simulink model "mcb_pmsm_foc_hall_f28379d_state_indicator"  (R2023b)
settings: Solver=FixedStepDiscrete  StartTime=0.0  StopTime=8  RelTol=1e-3  EnableMultiTasking=on
InitFcn:
  | mcb_pmsm_foc_hall_f28379d_data;
model workspace (MAT data in the model file):
  encoderResolution = 2000
  hallOffset = '0.5'
  indexOffset = 850
  polePairs = '4'
values from neighbouring files (symbols this model uses):
  dataType = 'single'    [mcb_pmsm_foc_hall_f28069m_data.m]    (also in mcb_pmsm_foc_hall_f28379d_data.m)
  inverter = mcb_SetInverterParameters('DRV8312-C2-KIT')    [mcb_pmsm_foc_hall_f28069m_data.m]    (also in mcb_pmsm_foc_hall_f28379d_data.m = mcb_updateInverterParameters(pmsm,inverter,target))
  PI_params = mcb_SetControllerParameters(pmsm,inverter,PU_System,T_pwm,Ts,Ts_speed)    [mcb_pmsm_foc_hall_f28069m_data.m]    (also in mcb_pmsm_foc_hall_f28379d_data.m)
  pmsm = mcb_SetPMSMMotorParameters('BLY171D')    [mcb_pmsm_foc_hall_f28069m_data.m]    (also in mcb_pmsm_foc_hall_f28379d_data.m = mcb_SetPMSMMotorParameters('custom'))
  PU_System = mcb_SetPUSystem(pmsm,inverter)    [mcb_pmsm_foc_hall_f28069m_data.m]    (also in mcb_pmsm_foc_hall_f28379d_data.m)
  target = mcb_SetProcessorDetails('F28069M',PWM_frequency)    [mcb_pmsm_foc_hall_f28069m_data.m]    (also in mcb_pmsm_foc_hall_f28379d_data.m = mcb_SetProcessorDetails('F28379D',PWM_frequency))
  Ts = T_pwm    (= 5e-05)    [mcb_pmsm_foc_hall_f28069m_data.m]    (also in mcb_pmsm_foc_hall_f28379d_data.m)
  Ts_motor = T_pwm/2    (= 2.5e-05)    [mcb_pmsm_foc_hall_f28069m_data.m]    (also in mcb_pmsm_foc_hall_f28379d_data.m)
  Ts_simulink = T_pwm/2    (= 2.5e-05)    [mcb_pmsm_foc_hall_f28069m_data.m]    (also in mcb_pmsm_foc_hall_f28379d_data.m)
  Ts_speed = 10*Ts    (= 0.0005)    [mcb_pmsm_foc_hall_f28069m_data.m]    (also in mcb_pmsm_foc_hall_f28379d_data.m)
undefined symbols (not defined in the file or in its folder): DiscIntNeverNeededParam, Down, GPTRIP1SEL, GPTRIP2SEL, Ts_sensor, TZ1, TZ2, Up
libraries: simulink x37, mcbpositiondecoderlib x12, mcbcontrolslib x11, idelinklib_common x8, c280xlib x8, c2802xlib x7, svdschedulerlib x5, slpidlib x4, c2837xDlib x3, dspfdesign x2, cstblocks x2, svdutilitieslib x1
(part 1 of 4)
settings Model: ExtModeTrigDuration=8  Creator=The MathWorks, Inc.  LastModifiedBy=13571
settings SolverCC: AlgebraicLoopSolver=TrustRegion  AutoInsertRateTranBlk=on
settings DataIOCC: LimitDataPoints=on  SaveFormat=Array  SaveOutput=off  SaveTime=off  ReturnWorkspaceOutputs=off
settings OptimizationCC: DefaultParameterBehavior=Inlined  DefaultUnderspecifiedDataType=single  OptimizeBlockIOStorage=off  BufferReuse=off  ReuseModelBlockBuffer=off  GlobalBufferReuse=off  ExpressionFolding=off  ExpressionDepthLimit=2147483647  LocalBlockOutputs=off  InitFltsAndDblsToZero=on  NoFixptDivByZeroProtection=on  EfficientFloat2IntCast=on  EfficientMapNaN2IntZero=off  LifeSpan=Inf  MaxStackSize=512  OptimizeDataStoreBuffers=off  BusAssignmentInplaceUpdate=off  EfficientTunableParamExpr=on
settings DebuggingCC: ReadBeforeWriteMsg=DisableAll  WriteAfterWriteMsg=DisableAll  WriteAfterReadMsg=DisableAll  CheckSSInitialOutputMsg=off  SignalResolutionControl=TryResolveAllWithWarning  SolverPrmCheckMsg=warning  InheritedTsInSrcMsg=none  MultiTaskDSMMsg=none  MultiTaskCondExecSysMsg=none  TasksWithSamePriorityMsg=none  SigSpecEnsureSampleTimeMsg=none  IntegerOverflowMsg=none  ParameterPrecisionLossMsg=none  FcnCallInpInsideContextMsg=warning  UnconnectedInputMsg=warning  UnconnectedOutputMsg=warning  UnconnectedLineMsg=warning  AllowSymbolicDim=off  StateNameClashWarn=warning  PregeneratedLibrarySubsystemCodeDiagnostic=none  SFUnexpectedBacktrackingDiag=warning  SFNoUnconditionalDefaultTransitionDiag=warning  SFExecutionAtInitializationDiag=none  IntegerSaturationMsg=none  ArithmeticOperatorsInVariantConditions=warning
settings HardwareCC: ProdBitPerChar=16  ProdBitPerInt=16  ProdBitPerPointer=32  ProdBitPerSizeT=32  ProdBitPerPtrDiffT=32  ProdLargestAtomicInteger=Integer  ProdLargestAtomicFloat=None  ProdWordSize=16  ProdLongLongMode=on  ProdHWDeviceType=Texas Instruments->C2000  TargetBitPerChar=16  TargetBitPerInt=16  TargetBitPerPointer=16  TargetLargestAtomicInteger=Integer  TargetIntDivRoundTo=Zero  TargetEndianess=LittleEndian  TargetWordSize=16  TargetHWDeviceType=TI C2000
settings ModelReferenceCC: EnableRefExpFcnMdlSchedulingChecks=on  PropagateSignalLabelsOutOfModel=off
settings SFSimCC: SimUseLocalCustomCode=off  MATLABDynamicMemAlloc=off
settings RTWCC: Description=Embedded Coder  SystemTargetFile=ert.tlc  HardwareBoard=TI Delfino F28379D LaunchPad  TemplateMakefile=ert_default_tmf  GenerateReport=on  RTWUseLocalCustomCode=off  Toolchain=Texas Instruments Code Composer Studio (C2000)  IncludeHyperlinkInReport=on  GenerateTraceInfo=on  GenerateTraceReport=on  GenerateTraceReportSl=on  GenerateTraceReportSf=on  GenerateTraceReportEml=on  DLArmComputeVersion=19.05
settings CodeAppCC: IgnoreCustomStorageClasses=off  CustomSymbolStrType=$N$R$M  StateflowObjectComments=on  InternalIdentifier=Classic
settings ERTTargetCC: CodeReplacementLibrary=TI C28x  MultiwordLength=2048  ConvertIfToSwitch=off  SuppressUnreachableDefaultCases=off  MemSecPackage=tic2000demospkg
settings ConfigComp: CovMetricSettings=dw  CovSaveCumulativeToWorkspaceVar=on  CovSaveSingleToWorkspaceVar=on  CovExternalEMLEnable=off  CovSFcnEnable=off

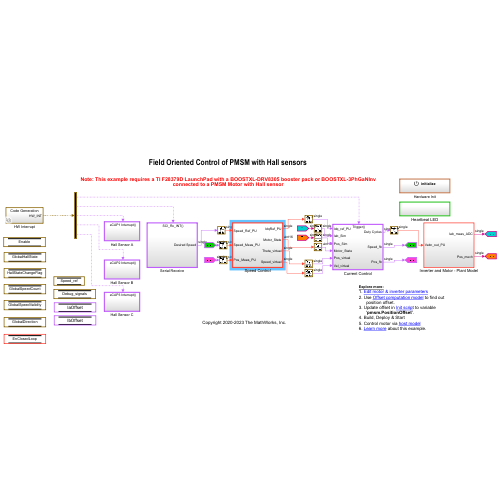
[thumbnail: Simulink's stored preview of the top-level diagram]
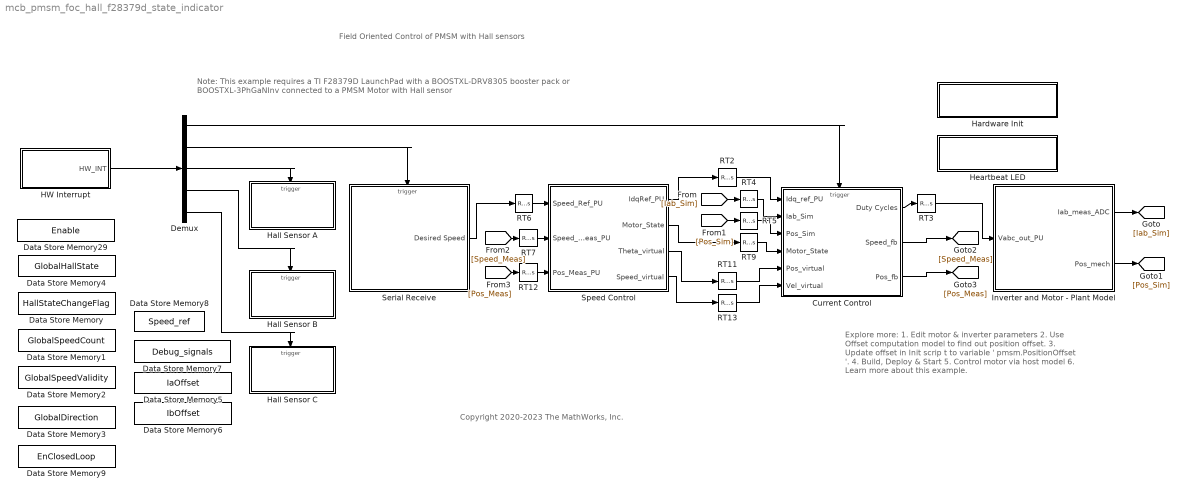
== system mcb_pmsm_foc_hall_f28379d_state_indicator ==
  note: Copyright 2020-2023 The MathWorks, Inc.
  note: Field Oriented Control of PMSM with Hall sensors
  note: Note: This example requires a TI F28379D LaunchPad with a BOOSTXL-DRV8305 booster pack or BOOSTXL-3PhGaNInv
      | connected to a PMSM Motor with Hall sensor
  note: Explore more:
      | 1. Edit motor & inverter parameters
      | 2. Use Offset computation model to find out position offset.
      | 3. Update offset in Init scrip t to variable ' pmsm.PositionOffset '.
      | 4. Build, Deploy & Start
      | 5. Control motor via host model
      | 6. Learn more about this example.
  Current Control : Subsystem
      settings: RTWSystemCode=Nonreusable function
  Data Store Memory : DataStoreMemory  DataStoreName=HallStateChangeFlag  ShowAdditionalParam=off
  Data Store Memory1 : DataStoreMemory  DataStoreName=GlobalSpeedCount  ShowAdditionalParam=off
  Data Store Memory2 : DataStoreMemory  DataStoreName=GlobalSpeedValidity  ShowAdditionalParam=off
  Data Store Memory29 : DataStoreMemory  DataStoreName=Enable  ShowAdditionalParam=off  OutDataTypeStr=boolean
  Data Store Memory3 : DataStoreMemory  DataStoreName=GlobalDirection  ShowAdditionalParam=off
  Data Store Memory4 : DataStoreMemory  DataStoreName=GlobalHallState  ShowAdditionalParam=off  OutDataTypeStr=uint32
  Data Store Memory5 : DataStoreMemory  DataStoreName=IaOffset  InitialValue=inverter.CtSensAOffset  ShowAdditionalParam=off
  Data Store Memory6 : DataStoreMemory  DataStoreName=IbOffset  InitialValue=inverter.CtSensBOffset  ShowAdditionalParam=off
  Data Store Memory7 : DataStoreMemory  DataStoreName=Debug_signals  ReadBeforeWriteMsg=warning  WriteAfterWriteMsg=warning  WriteAfterReadMsg=warning  InitialValue=5  ShowAdditionalParam=off  OutDataTypeStr=uint16
  Data Store Memory8 : DataStoreMemory  DataStoreName=Speed_ref  ReadBeforeWriteMsg=warning  WriteAfterWriteMsg=warning  WriteAfterReadMsg=warning  ShowAdditionalParam=off  OutDataTypeStr=dataType
  Data Store Memory9 : DataStoreMemory  DataStoreName=EnClosedLoop  WriteAfterWriteMsg=warning  ShowAdditionalParam=off
  Demux : Demux  Outputs=5
  HW Interrupt : Subsystem  Variant=on  VariantControlMode=sim codegen switching
  Hall Sensor A : Subsystem
  Hall Sensor B : Subsystem
  Hall Sensor C : Subsystem
  Hardware Init : Subsystem  TreatAsAtomicUnit=on
  Heartbeat LED : Subsystem  TreatAsAtomicUnit=on
  Inverter and Motor - Plant Model : Subsystem
  RT{2..5,9,11,13} (7 alike) : RateTransition  Deterministic=off
  RT12 : RateTransition  Deterministic=off  OutPortSampleTime=Ts_speed
  RT6 : RateTransition  Deterministic=off  OutPortSampleTime=Ts_speed
  RT7 : RateTransition  Deterministic=off  OutPortSampleTime=Ts_speed
  Serial Receive : Subsystem  SystemSampleTime=1e-3
  Speed Control : Subsystem  TreatAsAtomicUnit=on  SystemSampleTime=Ts_speed
  wires:
  [Iab_Sim] -> RT4/1
  Speed Control/1(IdqRef_PU) -> RT2/1
  [Pos_Sim] -> RT5/1
  RT2/1 -> Current Control/1(Idq_ref_PU)
  RT4/1 -> Current Control/2(Iab_Sim)
  RT5/1 -> Current Control/3(Pos_Sim)
  Current Control/1(Duty Cycles) -> RT3/1
  RT3/1 -> Inverter and Motor - Plant Model/1(Vabc_out_PU)
  Inverter and Motor - Plant Model/1(Iab_meas_ADC) -> [Iab_Sim]
  Inverter and Motor - Plant Model/2(Pos_mech) -> [Pos_Sim]
  Demux/2 -> Serial Receive/Trigger
  Demux/1 -> Current Control/Trigger
  HW Interrupt/1(HW_INT) -> Demux/1
  Demux/3 -> Hall Sensor A/Trigger
  Demux/4 -> Hall Sensor B/Trigger
  Demux/5 -> Hall Sensor C/Trigger
  Serial Receive/1(Desired Speed) -> RT6/1
  RT6/1 -> Speed Control/1(Speed_Ref_PU)
  RT7/1 -> Speed Control/2(Speed_Meas_PU)
  Speed Control/2(Motor_State) -> RT9/1
  RT9/1 -> Current Control/4(Motor_State)
  Speed Control/3(Theta_virtual) -> RT11/1
  RT11/1 -> Current Control/5(Pos_virtual)
  Current Control/2(Speed_fb) -> [Speed_Meas]
  [Speed_Meas] -> RT7/1
  Current Control/3(Pos_fb) -> [Pos_Meas]
  RT12/1 -> Speed Control/3(Pos_Meas_PU)
  [Pos_Meas] -> RT12/1
  Speed Control/4(Speed_virtual) -> RT13/1
  RT13/1 -> Current Control/6(Vel_virtual)

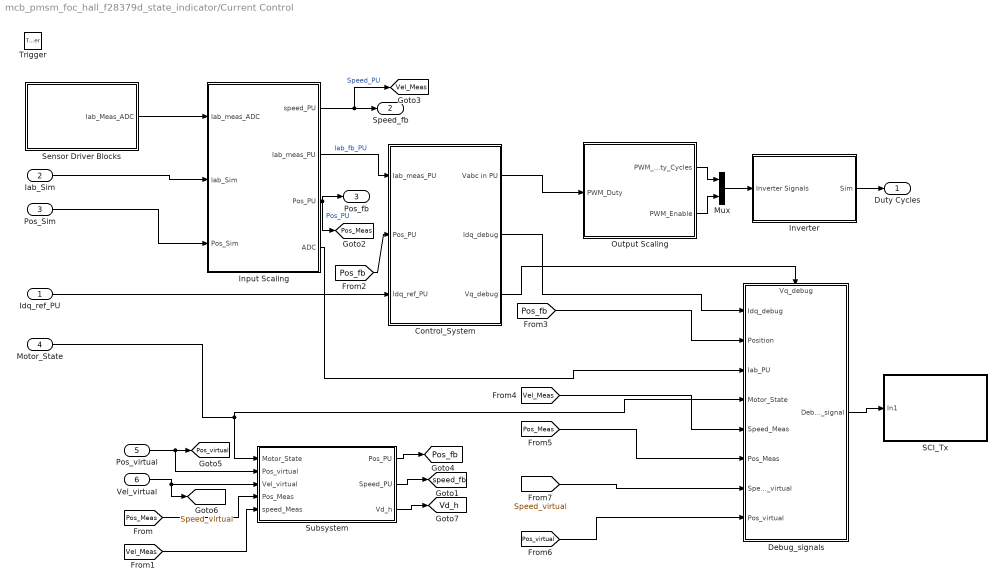
== system mcb_pmsm_foc_hall_f28379d_state_indicator/Current Control ==
  Idq_ref_PU : Inport
  Iab_Sim : Inport  Port=2
  Pos_Sim : Inport  Port=3
  Motor_State : Inport  Port=4
  Pos_virtual : Inport  Port=5
  Vel_virtual : Inport  Port=6
  Trigger : TriggerPort  TriggerType=function-call  VariantControl=Variant  PortDimensions=1
  Control_System : Subsystem
  Debug_signals : Subsystem
      settings: PortSchema="{\"entries\":[{\"content\":{\"sides\":[{\"content\":{\"connectorIds\":[\"In1\",\"In2\",\"In3\",\"In4\",\"In5\",\"In6\",\"In7\",\"In8\"]},\"type\":\"ConnectorPlacement.EquallySpacedRectSide\",\"uuid\":\"67483f5e-56e2-47cf-8de8-9bd8ec9baffc\"},{\"content\":{\"connectorIds\":[\"Out1\"],\"side\":\"RIGHT\"},\"type\":\"ConnectorPlacement.EquallySpacedRectSide\",\"uuid\":\"d939e1f4-c08d-487b-bf48-149d22cc5739\"},{\"content\":{\"connectorIds\":[\"In9\"],\"side\":\"TOP\"},\"type\":\"ConnectorPlacement.EquallySpacedRectSide\",\"uuid\":\"48db4f3d-d2f9-4eaf-b7c1-a7fd508ed9fd\"}]},\"type\":\"ConnectorPlacement.EquallySpacedConnector\",\"uuid\":\"f00bd8a8-e348-4ac0-9697-8b50afb0be3d\"}],\"packageUris\":[\"http://schema.mathworks.com/mf0/Connector/R2020b\"],\"version\":\"1.0\"}"
  Input Scaling : Subsystem  Variant=on  VariantControlMode=sim codegen switching  VariantControl=Variant1  PropagateVariantConditions=on
  Inverter : Subsystem  Variant=on  VariantControlMode=sim codegen switching
  Mux : Mux  Inputs=2
  Output Scaling : Subsystem
  SCI_Tx : Subsystem  Variant=on  VariantControlMode=sim codegen switching
  Sensor Driver Blocks : Subsystem  Variant=on  VariantControlMode=sim codegen switching
  Subsystem : Subsystem
  Duty Cycles : Outport  InitialOutput=0  VectorParamsAs1DForOutWhenUnconnected=off
  Speed_fb : Outport  Port=2  InitialOutput=0  VectorParamsAs1DForOutWhenUnconnected=off
  Pos_fb : Outport  Port=3  InitialOutput=0  VectorParamsAs1DForOutWhenUnconnected=off
  tag scope: Pos_Meas=global, Pos_fb=global, Pos_virtual=global, Speed_virtual=global, Vd_h=global, Vel_Meas=global, speed_fb=global
  wires:
  Control_System/1(Vabc in PU) -> Output Scaling/1(PWM_Duty)
  Idq_ref_PU/1 -> Control_System/3(Idq_ref_PU)
  Input Scaling/2(Iab_meas_PU) -> Control_System/1(Iab_meas_PU)  "Iab_fb_PU"
  Sensor Driver Blocks/1(Iab_Meas_ADC) -> Input Scaling/1(Iab_meas_ADC)
  Iab_Sim/1 -> Input Scaling/2(Iab_Sim)
  Pos_Sim/1 -> Input Scaling/3(Pos_Sim)
  Inverter/1(Sim) -> Duty Cycles/1
  Debug_signals/1(Debug_signal) -> SCI_Tx/1(In1)
  Mux/1 -> Inverter/1(Inverter Signals)
  Output Scaling/2(PWM_Enable) -> Mux/2
  Output Scaling/1(PWM_Duty_Cycles) -> Mux/1
  Control_System/2(Idq_debug) -> Debug_signals/1(Idq_debug)
  Input Scaling/4(ADC) -> Debug_signals/3(Iab_PU)
  Motor_State/1 -> Subsystem/1(Motor_State), Debug_signals/4(Motor_State)
  Subsystem/1(Pos_PU) -> [Pos_fb]
  Input Scaling/3(Pos_PU) -> Pos_fb/1, [Pos_Meas]  "Pos_PU"
  [Pos_Meas] -> Subsystem/4(Pos_Meas)
  [Vel_Meas] -> Subsystem/5(speed_Meas)
  Input Scaling/1(speed_PU) -> Speed_fb/1, [Vel_Meas]  "Speed_PU"
  [Pos_fb] -> Debug_signals/2(Position)
  [Vel_Meas] -> Debug_signals/5(Speed_Meas)
  [Pos_Meas] -> Debug_signals/6(Pos_Meas)
  Pos_virtual/1 -> Subsystem/2(Pos_virtual), [Pos_virtual]
  [Pos_virtual] -> Debug_signals/8(Pos_virtual)
  [Speed_virtual] -> Debug_signals/7(Speed_virtual)
  Subsystem/2(Speed_PU) -> [speed_fb]
  Vel_virtual/1 -> [Speed_virtual], Subsystem/3(Vel_virtual)
  Control_System/3(Vq_debug) -> Debug_signals/9(Vq_debug)
  Subsystem/3(Vd_h) -> [Vd_h]
  [Pos_fb] -> Control_System/2(Pos_PU)

== system mcb_pmsm_foc_hall_f28379d_state_indicator/HW Interrupt ==
  Code Generation : Subsystem  VariantControl=(codegen)
  Simulation : Subsystem  VariantControl=(sim)
  HW_INT : Outport  VectorParamsAs1DForOutWhenUnconnected=off  OutputFunctionCall=on

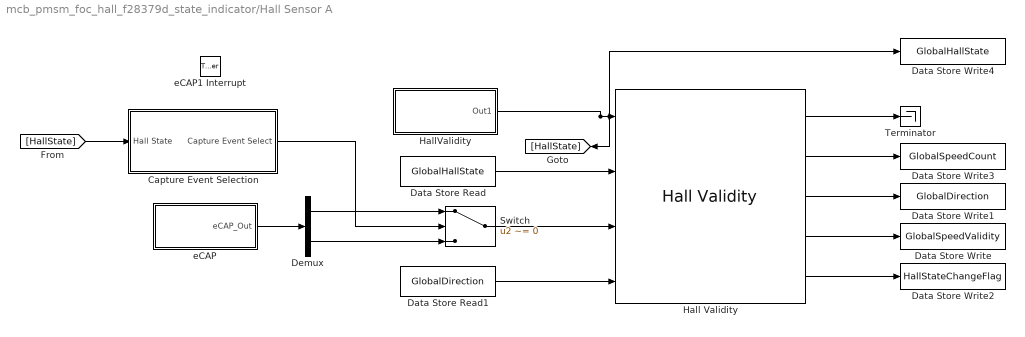
== system mcb_pmsm_foc_hall_f28379d_state_indicator/Hall Sensor A ==
  eCAP1 Interrupt : TriggerPort  TriggerType=function-call  VariantControl=Variant
  Capture Event Selection : Subsystem
  Data Store Read : DataStoreRead  Priority=1  DataStoreName=GlobalHallState  IndexOptions=Index vector (dialog)  Indices=1  OutputSizes=1
  Data Store Read1 : DataStoreRead  DataStoreName=GlobalDirection  IndexOptions=Index vector (dialog)  Indices=1  OutputSizes=1
  Data Store Write : DataStoreWrite  DataStoreName=GlobalSpeedValidity  IndexOptions=Index vector (dialog)  Indices=1  OutputSizes=1
  Data Store Write1 : DataStoreWrite  DataStoreName=GlobalDirection  IndexOptions=Index vector (dialog)  Indices=1  OutputSizes=1
  Data Store Write2 : DataStoreWrite  DataStoreName=HallStateChangeFlag  IndexOptions=Index vector (dialog)  Indices=1  OutputSizes=1
  Data Store Write3 : DataStoreWrite  DataStoreName=GlobalSpeedCount  IndexOptions=Index vector (dialog)  Indices=1  OutputSizes=1
  Data Store Write4 : DataStoreWrite  Priority=2  DataStoreName=GlobalHallState  IndexOptions=Index vector (dialog)  Indices=1  OutputSizes=1
  Demux : Demux  Outputs=2
  Hall Validity : mcbpositiondecoderlib/Hall Validity  hallSequence=ABC  sequence=[5,4,6,2,3,1]  CounterSize=32 bits
  HallValidity : Subsystem  Variant=on  VariantControlMode=sim codegen switching
  Switch : Switch  Criteria=u2 ~= 0  SaturateOnIntegerOverflow=off  InputSameDT=off
  Terminator : Terminator
  eCAP : Subsystem  Variant=on  VariantControlMode=sim codegen switching
  wires:
  Hall Validity/3 -> Data Store Write1/1
  Hall Validity/5 -> Data Store Write2/1
  Hall Validity/4 -> Data Store Write/1
  Data Store Read/1 -> Hall Validity/2
  Data Store Read1/1 -> Hall Validity/4
  Switch/1 -> Hall Validity/3
  Hall Validity/2 -> Data Store Write3/1
  Demux/2 -> Switch/3
  Demux/1 -> Switch/1
  Hall Validity/1 -> Terminator/1
  Capture Event Selection/1(Capture Event Select) -> Switch/2
  [HallState] -> Capture Event Selection/1(Hall State)
  eCAP/1(eCAP_Out) -> Demux/1
  HallValidity/1(Out1) -> [HallState], Data Store Write4/1, Hall Validity/1

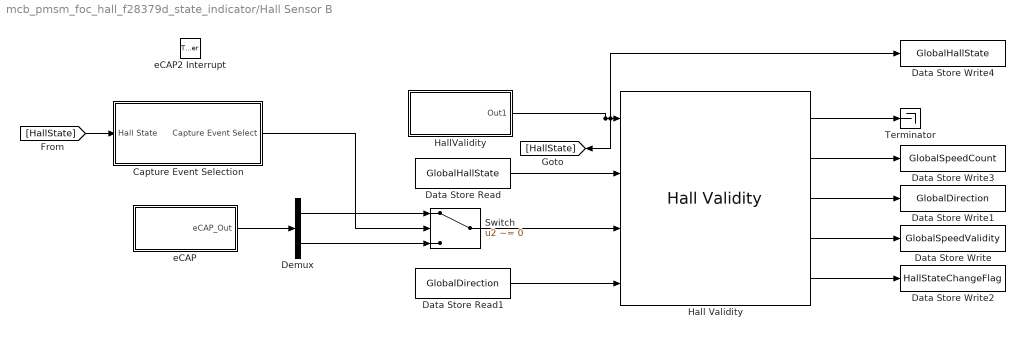
== system mcb_pmsm_foc_hall_f28379d_state_indicator/Hall Sensor B ==
  eCAP2 Interrupt : TriggerPort  TriggerType=function-call  VariantControl=Variant
  Capture Event Selection : Subsystem
  Data Store Read : DataStoreRead  Priority=1  DataStoreName=GlobalHallState  IndexOptions=Index vector (dialog)  Indices=1  OutputSizes=1
  Data Store Read1 : DataStoreRead  DataStoreName=GlobalDirection  IndexOptions=Index vector (dialog)  Indices=1  OutputSizes=1
  Data Store Write : DataStoreWrite  DataStoreName=GlobalSpeedValidity  IndexOptions=Index vector (dialog)  Indices=1  OutputSizes=1
  Data Store Write1 : DataStoreWrite  DataStoreName=GlobalDirection  IndexOptions=Index vector (dialog)  Indices=1  OutputSizes=1
  Data Store Write2 : DataStoreWrite  DataStoreName=HallStateChangeFlag  IndexOptions=Index vector (dialog)  Indices=1  OutputSizes=1
  Data Store Write3 : DataStoreWrite  DataStoreName=GlobalSpeedCount  IndexOptions=Index vector (dialog)  Indices=1  OutputSizes=1
  Data Store Write4 : DataStoreWrite  Priority=2  DataStoreName=GlobalHallState  IndexOptions=Index vector (dialog)  Indices=1  OutputSizes=1
  Demux : Demux  Outputs=2
  Hall Validity : mcbpositiondecoderlib/Hall Validity  hallSequence=ABC  sequence=[5,4,6,2,3,1]  CounterSize=32 bits
  HallValidity : Subsystem  Variant=on  VariantControlMode=sim codegen switching
  Switch : Switch  Criteria=u2 ~= 0  Threshold=3  SaturateOnIntegerOverflow=off  InputSameDT=off
  Terminator : Terminator
  eCAP : Subsystem  Variant=on  VariantControlMode=sim codegen switching
  wires:
  Hall Validity/3 -> Data Store Write1/1
  Hall Validity/5 -> Data Store Write2/1
  Hall Validity/4 -> Data Store Write/1
  Data Store Read1/1 -> Hall Validity/4
  Hall Validity/2 -> Data Store Write3/1
  Data Store Read/1 -> Hall Validity/2
  Demux/1 -> Switch/1
  Demux/2 -> Switch/3
  Switch/1 -> Hall Validity/3
  Hall Validity/1 -> Terminator/1
  [HallState] -> Capture Event Selection/1(Hall State)
  Capture Event Selection/1(Capture Event Select) -> Switch/2
  eCAP/1(eCAP_Out) -> Demux/1
  HallValidity/1(Out1) -> [HallState], Data Store Write4/1, Hall Validity/1

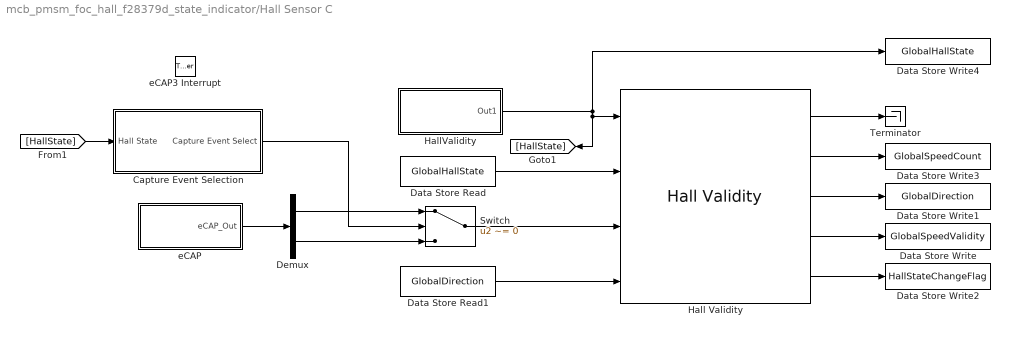
== system mcb_pmsm_foc_hall_f28379d_state_indicator/Hall Sensor C ==
  eCAP3 Interrupt : TriggerPort  TriggerType=function-call  VariantControl=Variant
  Capture Event Selection : Subsystem
  Data Store Read : DataStoreRead  Priority=1  DataStoreName=GlobalHallState  IndexOptions=Index vector (dialog)  Indices=1  OutputSizes=1
  Data Store Read1 : DataStoreRead  DataStoreName=GlobalDirection  IndexOptions=Index vector (dialog)  Indices=1  OutputSizes=1
  Data Store Write : DataStoreWrite  DataStoreName=GlobalSpeedValidity  IndexOptions=Index vector (dialog)  Indices=1  OutputSizes=1
  Data Store Write1 : DataStoreWrite  DataStoreName=GlobalDirection  IndexOptions=Index vector (dialog)  Indices=1  OutputSizes=1
  Data Store Write2 : DataStoreWrite  DataStoreName=HallStateChangeFlag  IndexOptions=Index vector (dialog)  Indices=1  OutputSizes=1
  Data Store Write3 : DataStoreWrite  DataStoreName=GlobalSpeedCount  IndexOptions=Index vector (dialog)  Indices=1  OutputSizes=1
  Data Store Write4 : DataStoreWrite  Priority=2  DataStoreName=GlobalHallState  IndexOptions=Index vector (dialog)  Indices=1  OutputSizes=1
  Demux : Demux  Outputs=2
  Hall Validity : mcbpositiondecoderlib/Hall Validity  hallSequence=ABC  sequence=[5,4,6,2,3,1]  CounterSize=32 bits
  HallValidity : Subsystem  Variant=on  VariantControlMode=sim codegen switching
  Switch : Switch  Criteria=u2 ~= 0  Threshold=3  SaturateOnIntegerOverflow=off  InputSameDT=off
  Terminator : Terminator
  eCAP : Subsystem  Variant=on  VariantControlMode=sim codegen switching
  wires:
  Hall Validity/3 -> Data Store Write1/1
  Hall Validity/5 -> Data Store Write2/1
  Hall Validity/4 -> Data Store Write/1
  Data Store Read1/1 -> Hall Validity/4
  Hall Validity/2 -> Data Store Write3/1
  Data Store Read/1 -> Hall Validity/2
  Demux/1 -> Switch/1
  Demux/2 -> Switch/3
  Switch/1 -> Hall Validity/3
  Hall Validity/1 -> Terminator/1
  [HallState] -> Capture Event Selection/1(Hall State)
  Capture Event Selection/1(Capture Event Select) -> Switch/2
  eCAP/1(eCAP_Out) -> Demux/1
  HallValidity/1(Out1) -> Data Store Write4/1, Hall Validity/1, [HallState]

== system mcb_pmsm_foc_hall_f28379d_state_indicator/Hardware Init ==
  6PWM_Mode : Constant  Priority=1000  Value=0x3A16  OutDataTypeStr=uint16  SampleTime=-1
  ADC_Gain_Setting : Constant  Priority=1000  Value=inverter.SPI_Gain_Setting  OutDataTypeStr=uint16  SampleTime=-1
  Event Listener : EventListener  DisableCoverage=on  EventName=reset
  Mux : Mux  Inputs=2
  Variant Subsystem : Subsystem  Variant=on  VariantControlMode=sim codegen switching
  wires:
  6PWM_Mode/1 -> Mux/1
  ADC_Gain_Setting/1 -> Mux/2
  Mux/1 -> Variant Subsystem/1(In1)

== system mcb_pmsm_foc_hall_f28379d_state_indicator/Heartbeat LED ==
  note: Heartbeat LED 1HZ
  Heartbeat LED : Subsystem  Variant=on  VariantControlMode=sim codegen switching
  RED_LED : Constant  OutDataTypeStr=uint16  SampleTime=0.5
  wires:
  RED_LED/1 -> Heartbeat LED/1(In1)

== system mcb_pmsm_foc_hall_f28379d_state_indicator/Inverter and Motor - Plant Model ==
  Vabc_out_PU : Inport
  Codegeneration : Subsystem
  Simulation : Subsystem
  Variant Sink : VariantSink  VariantControlMode=sim codegen switching
  Variant Source : VariantSource  VariantControlMode=sim codegen switching
  Variant Source1 : VariantSource  VariantControlMode=sim codegen switching
  Iab_meas_ADC : Outport  VectorParamsAs1DForOutWhenUnconnected=off
  Pos_mech : Outport  Port=2  VectorParamsAs1DForOutWhenUnconnected=off
  wires:
  Codegeneration/2(Pos_fb_Sim) -> Variant Source1/1
  Codegeneration/1(Iab_fb_Sim) -> Variant Source/1
  Variant Source1/1 -> Pos_mech/1
  Variant Sink/1 -> Codegeneration/1(Duty_Cycles)
  Variant Source/1 -> Iab_meas_ADC/1
  Simulation/1(Iab_fb_Sim) -> Variant Source/2
  Variant Sink/2 -> Simulation/1(Duty_Cycles)
  Simulation/2(Pos_fb_Sim) -> Variant Source1/2
  Vabc_out_PU/1 -> Variant Sink/1

== system mcb_pmsm_foc_hall_f28379d_state_indicator/Serial Receive ==
  SCI_Rx_INT : TriggerPort  TriggerType=function-call  VariantControl=Variant
  Data Store Write : DataStoreWrite  DataStoreName=Enable  IndexOptions=Index vector (dialog)  Indices=1  OutputSizes=1
  Data Store Write1 : DataStoreWrite  DataStoreName=Speed_ref  IndexOptions=Index vector (dialog)  Indices=1  OutputSizes=1
  Data Store Write2 : DataStoreWrite  DataStoreName=Debug_signals  IndexOptions=Index vector (dialog)  Indices=1  OutputSizes=1
  Data_Conditioning_Rx : Subsystem  Variant=on
  SCI_Rx : Subsystem  Variant=on  VariantControlMode=sim codegen switching
  unParse : Subsystem
  Desired Speed : Outport  VectorParamsAs1DForOutWhenUnconnected=off
  wires:
  unParse/2(Debug_signals) -> Data Store Write2/1
  Data_Conditioning_Rx/2(Out2) -> unParse/1(Data)
  SCI_Rx/1(Data) -> Data_Conditioning_Rx/1(In1)
  unParse/1(Enable_PWM) -> Data Store Write/1
  Data_Conditioning_Rx/1(Desired Speed) -> Desired Speed/1, Data Store Write1/1

== system mcb_pmsm_foc_hall_f28379d_state_indicator/Speed Control ==
  Speed_Ref_PU : Inport
  Speed_Meas_PU : Inport  Port=2
  Pos_Meas_PU : Inport  Port=3
  Id_ref : Constant  Value=0  OutDataTypeStr=dataType  SampleTime=Ts_speed
  Mux1 : Mux  Inputs=2
  PI_Controller_Speed : Subsystem  Commented=on
  PI_Controller_Speed2 : Subsystem
  Speed_Ref_Selector : Subsystem
  IdqRef_PU : Outport  VectorParamsAs1DForOutWhenUnconnected=off
  Motor_State : Outport  Port=2  VectorParamsAs1DForOutWhenUnconnected=off
  Theta_virtual : Outport  Port=3  VectorParamsAs1DForOutWhenUnconnected=off
  Speed_virtual : Outport  Port=4  VectorParamsAs1DForOutWhenUnconnected=off
  wires:
  Mux1/1 -> IdqRef_PU/1
  Speed_Meas_PU/1 -> PI_Controller_Speed2/2(N_fb), Speed_Ref_Selector/2(Speed_Ref_Open)  "Speed_fb"
  Speed_Ref_PU/1 -> Speed_Ref_Selector/1(Speed_Ref_In)
  Id_ref/1 -> Mux1/1
  Speed_Ref_Selector/1(Speed_Ref_PU) -> PI_Controller_Speed2/1(N_ref)  "Speed_Ref"
  PI_Controller_Speed2/1(Iq_ref) -> Mux1/2
  Pos_Meas_PU/1 -> PI_Controller_Speed2/3(Theta_Meas)
  PI_Controller_Speed2/2(theta_virtual) -> Theta_virtual/1
  PI_Controller_Speed2/3(speed_virtual) -> Speed_virtual/1
  PI_Controller_Speed2/4(Motor_State) -> Motor_State/1

== system mcb_pmsm_foc_hall_f28379d_state_indicator/Current Control/Control_System ==
  Iab_meas_PU : Inport
  Pos_PU : Inport  Port=2
  Idq_ref_PU : Inport  Port=3
  Clarke Transform : mcbcontrolslib/Clarke Transform  VariantControl=Variant2  PhaseInput=Two inputs  EnPowerInv=off
  Current_Controllers : Subsystem
  Demux : Demux  Outputs=2
  Inverse Park Transform : mcbcontrolslib/Inverse Park Transform  PhaseInput=Two inputs  AxisAlignment=D-axis  ThetaInput=Electrical position  AngleInput=Per-unit  N_points=1024
  Mux1 : Mux  Inputs=3
  Park Transform : mcbcontrolslib/Park Transform  PhaseInput=Two inputs  AxisAlignment=D-axis  ThetaInput=Electrical position  AngleInput=Per-unit  N_points=1024
  Space Vector Generator : mcbcontrolslib/PWM Reference Generator  inSignal=Valphabeta  modType=SVM: space vector modulation
  Sum : Sum  Inputs=|++
  提取基频信号 : Subsystem
  Vabc in PU : Outport  VectorParamsAs1DForOutWhenUnconnected=off
  Idq_debug : Outport  Port=2  VectorParamsAs1DForOutWhenUnconnected=off
  Vq_debug : Outport  Port=3  VectorParamsAs1DForOutWhenUnconnected=off
  wires:
  Mux1/1 -> Vabc in PU/1
  Space Vector Generator/3 -> Mux1/3
  Idq_ref_PU/1 -> Current_Controllers/3(Idq_ref_PU)
  Iab_meas_PU/1 -> Demux/1
  Demux/2 -> Clarke Transform/2
  Space Vector Generator/1 -> Mux1/1
  Demux/1 -> Clarke Transform/1
  Inverse Park Transform/2 -> Space Vector Generator/2
  Space Vector Generator/2 -> Mux1/2
  Clarke Transform/1 -> Park Transform/1
  Pos_PU/1 -> Inverse Park Transform/3, Park Transform/3
  Clarke Transform/2 -> Park Transform/2
  Current_Controllers/2(Vq_ref) -> Vq_debug/1, Inverse Park Transform/2
  Inverse Park Transform/1 -> Space Vector Generator/1
  Current_Controllers/3(Idq) -> Idq_debug/1
  Park Transform/1 -> 提取基频信号/1(id)
  Park Transform/2 -> 提取基频信号/2(iq)
  Current_Controllers/1(Vd_ref) -> Sum/2
  Sum/1 -> Inverse Park Transform/1
  [Vd_h] -> Sum/1
  提取基频信号/1(idf) -> Current_Controllers/1(Id)
  提取基频信号/2(iqf) -> Current_Controllers/2(Iq)

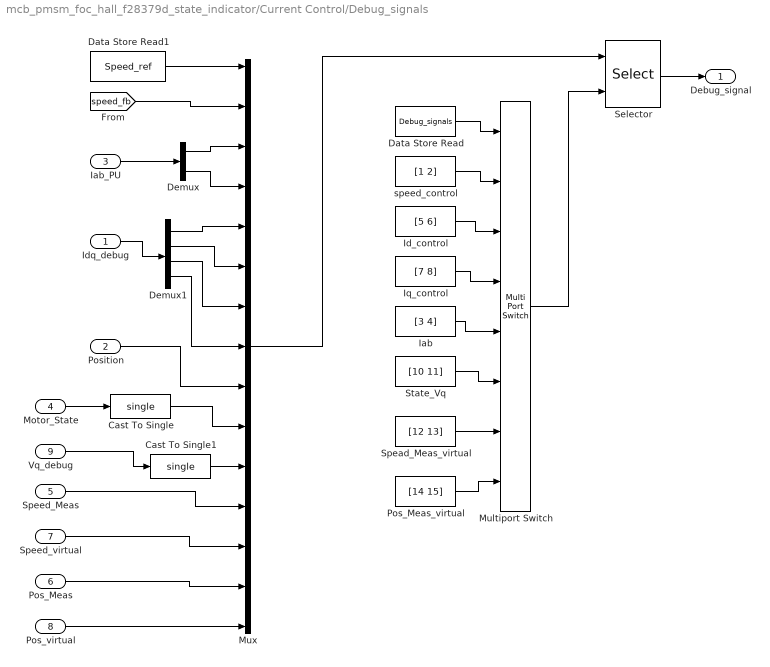
== system mcb_pmsm_foc_hall_f28379d_state_indicator/Current Control/Debug_signals ==
  Idq_debug : Inport
  Position : Inport  Port=2
  Iab_PU : Inport  Port=3
  Motor_State : Inport  Port=4
  Speed_Meas : Inport  Port=5
  Pos_Meas : Inport  Port=6
  Speed_virtual : Inport  Port=7
  Pos_virtual : Inport  Port=8
  Vq_debug : Inport  Port=9
  Cast To Single : DataTypeConversion  OutDataTypeStr=single  SaturateOnIntegerOverflow=off  RndMeth=Floor
  Cast To Single1 : DataTypeConversion  OutDataTypeStr=single  SaturateOnIntegerOverflow=off  RndMeth=Floor
  Data Store Read : DataStoreRead  DataStoreName=Debug_signals  IndexOptions=Index vector (dialog)  Indices=1  OutputSizes=1
  Data Store Read1 : DataStoreRead  DataStoreName=Speed_ref  IndexOptions=Index vector (dialog)  Indices=1  OutputSizes=1
  Demux : Demux  Outputs=2
  Demux1 : Demux
  Iab : Constant  Value=[3 4]  OutDataTypeStr=uint16  SampleTime=-1
  Id_control : Constant  Value=[5 6]  OutDataTypeStr=uint16  SampleTime=-1
  Iq_control : Constant  Value=[7 8]  OutDataTypeStr=uint16  SampleTime=-1
  Multiport Switch : MultiPortSwitch  Inputs=7  DiagnosticForDefault=Warning  OutDataTypeStr=uint16  RndMeth=Simplest  SaturateOnIntegerOverflow=off  InputSameDT=off
  Mux : Mux  Inputs=15
  Pos_Meas_virtual : Constant  Value=[14 15]  OutDataTypeStr=uint16  SampleTime=-1
  Selector : Selector  InputPortWidth=15  IndexOptions=Index vector (port)  Indices=[1 3]  OutputSizes=1
  Spead_Meas_virtual : Constant  Value=[12 13]  OutDataTypeStr=uint16  SampleTime=-1
  State_Vq : Constant  Value=[10 11]  OutDataTypeStr=uint16  SampleTime=-1
  speed_control : Constant  Value=[1 2]  OutDataTypeStr=uint16  SampleTime=-1
  Debug_signal : Outport
  wires:
  speed_control/1 -> Multiport Switch/2
  Id_control/1 -> Multiport Switch/3
  Iq_control/1 -> Multiport Switch/4
  Iab/1 -> Multiport Switch/5
  State_Vq/1 -> Multiport Switch/6
  Multiport Switch/1 -> Selector/2
  Data Store Read/1 -> Multiport Switch/1
  Selector/1 -> Debug_signal/1
  Iab_PU/1 -> Demux/1
  Demux/1 -> Mux/3
  Demux/2 -> Mux/4
  Demux1/1 -> Mux/5
  Demux1/2 -> Mux/6
  Demux1/3 -> Mux/7
  Demux1/4 -> Mux/8
  Idq_debug/1 -> Demux1/1
  Mux/1 -> Selector/1
  [speed_fb] -> Mux/2
  Data Store Read1/1 -> Mux/1
  Position/1 -> Mux/9
  Cast To Single/1 -> Mux/10
  Motor_State/1 -> Cast To Single/1
  Speed_Meas/1 -> Mux/12
  Pos_Meas/1 -> Mux/14
  Speed_virtual/1 -> Mux/13
  Pos_virtual/1 -> Mux/15
  Spead_Meas_virtual/1 -> Multiport Switch/7
  Pos_Meas_virtual/1 -> Multiport Switch/8
  Vq_debug/1 -> Cast To Single1/1
  Cast To Single1/1 -> Mux/11

== system mcb_pmsm_foc_hall_f28379d_state_indicator/Current Control/Input Scaling ==
  Iab_meas_ADC : Inport
  Iab_Sim : Inport  Port=2
  Pos_Sim : Inport  Port=3
  Read_Sensor (codegen) : Subsystem  VariantControl=(codegen)
  Read_Sensor (sim) : Subsystem  VariantControl=(sim)
  speed_PU : Outport  InitialOutput=0  VectorParamsAs1DForOutWhenUnconnected=off
  Iab_meas_PU : Outport  Port=2  VectorParamsAs1DForOutWhenUnconnected=off
  Pos_PU : Outport  Port=3  InitialOutput=0  VectorParamsAs1DForOutWhenUnconnected=off
  ADC : Outport  Port=4  InitialOutput=0  VectorParamsAs1DForOutWhenUnconnected=off

== system mcb_pmsm_foc_hall_f28379d_state_indicator/Current Control/Inverter ==
  Inverter Signals : Inport
  Code Generation : Subsystem  VariantControl=(codegen)
  Simulation : Subsystem  VariantControl=(sim)
  Sim : Outport  VectorParamsAs1DForOutWhenUnconnected=off

== system mcb_pmsm_foc_hall_f28379d_state_indicator/Current Control/Output Scaling ==
  PWM_Duty : Inport
  Constant : Constant  Value=0.5  OutDataTypeStr=dataType
  Data Type Conversion : DataTypeConversion  OutDataTypeStr=dataType  SaturateOnIntegerOverflow=off  RndMeth=Floor
  Enable : DataStoreRead  DataStoreName=Enable  IndexOptions=Index vector (dialog)  Indices=1  OutputSizes=1
  Gain : Gain  Gain=0.5  OutDataTypeStr=dataType  RndMeth=Simplest
  Sum : Sum  Inputs=|++
  PWM_Duty_Cycles : Outport
  PWM_Enable : Outport  Port=2
  wires:
  Gain/1 -> Sum/1
  Sum/1 -> PWM_Duty_Cycles/1  "PWM_Duty_Cycles"
  Constant/1 -> Sum/2
  Enable/1 -> Data Type Conversion/1
  PWM_Duty/1 -> Gain/1
  Data Type Conversion/1 -> PWM_Enable/1

== system mcb_pmsm_foc_hall_f28379d_state_indicator/Current Control/SCI_Tx ==
  In1 : Inport
  Code Generation : Subsystem  VariantControl=(codegen)
  Simulation : Subsystem  VariantControl=(sim)

== system mcb_pmsm_foc_hall_f28379d_state_indicator/Current Control/Sensor Driver Blocks ==
  Sensor Driver Blocks (codegen) : Subsystem  VariantControl=(codegen)
  Sensor Driver Blocks (sim) : Subsystem  VariantControl=(sim)
  Iab_Meas_ADC : Outport

== system mcb_pmsm_foc_hall_f28379d_state_indicator/Current Control/Subsystem ==
  Motor_State : Inport
  Pos_virtual : Inport  Port=2
  Vel_virtual : Inport  Port=3
  Pos_Meas : Inport  Port=4
  speed_Meas : Inport  Port=5
  If Action Subsystem : Subsystem  TreatAsAtomicUnit=on
  If Action Subsystem1 : Subsystem  TreatAsAtomicUnit=on
  If Action Subsystem2 : Subsystem  TreatAsAtomicUnit=on
  If Action Subsystem3 : Subsystem  TreatAsAtomicUnit=on
  Merge : Merge  Inputs=4
  Merge1 : Merge  Inputs=4
  Merge2 : Merge  Inputs=4
  Switch Case : SwitchCase  CaseConditions={1,2,3,4}  ShowDefaultCase=off
  Pos_PU : Outport  InitialOutput=0  VectorParamsAs1DForOutWhenUnconnected=off
  Speed_PU : Outport  Port=2  InitialOutput=0  VectorParamsAs1DForOutWhenUnconnected=off
  Vd_h : Outport  Port=3  InitialOutput=0  VectorParamsAs1DForOutWhenUnconnected=off
  wires:
  Merge1/1 -> Speed_PU/1
  If Action Subsystem/2(Speed_PU) -> Merge1/1
  Motor_State/1 -> Switch Case/1
  If Action Subsystem/1(Pos_PU) -> Merge/1
  Merge/1 -> Pos_PU/1
  Pos_Meas/1 -> If Action Subsystem1/1(Pos_Meas)
  speed_Meas/1 -> If Action Subsystem1/2(speed_Meas)
  Vel_virtual/1 -> If Action Subsystem3/2(Vel_virtual), If Action Subsystem2/2(Vel_virtual), If Action Subsystem/2(Vel_virtual)
  If Action Subsystem/3(Vd_h) -> Merge2/1
  Merge2/1 -> Vd_h/1
  Switch Case/1 -> If Action Subsystem/Action
  Switch Case/2 -> If Action Subsystem2/Action
  Switch Case/3 -> If Action Subsystem3/Action
  Pos_virtual/1 -> If Action Subsystem/1(Pos_virtual), If Action Subsystem2/1(Pos_virtual), If Action Subsystem3/1(Pos_virtual)
  Switch Case/4 -> If Action Subsystem1/Action
  If Action Subsystem2/1(Pos_PU) -> Merge/2
  If Action Subsystem3/1(Pos_PU) -> Merge/3
  If Action Subsystem1/1(Pos_PU) -> Merge/4
  If Action Subsystem2/2(Speed_PU) -> Merge1/2
  If Action Subsystem3/2(Speed_PU) -> Merge1/3
  If Action Subsystem1/2(Speed_PU) -> Merge1/4
  If Action Subsystem2/3(Vd_h) -> Merge2/2
  If Action Subsystem3/3(Vd_h) -> Merge2/3
  If Action Subsystem1/3(Vd_h) -> Merge2/4

== system mcb_pmsm_foc_hall_f28379d_state_indicator/HW Interrupt/Code Generation ==
  HWI_ADCB1_INT : svdschedulerlib/Hardware Interrupt v2  ISRGroup=ADC - Analog to Digital Converter  ISRName=ADCA1_INT  ISRNumber=32  NumEventsToServe=1  EventsList={'on','EOC event','1';'off','Overflow event','2';'off','Custom event','3'}  SelectedEvents={'event1'}  TaskPriority=30  DisablePreemption=off  ClearInterruptFlagsAtEndOfEvent=on  InterruptDefinitionFile=$(TARGET_ROOT)/registry/interrupts/F2837xS_interrupts.xml  HardwareBoard=F2837x  EnableSimPort=off
      settings: LibrarySourceBlock=c2000lib/Scheduling/Hardware Interrupt
  HWI_ECAP1_INT : svdschedulerlib/Hardware Interrupt v2  ISRGroup=ADC - Analog to Digital Converter  ISRName=ADCA1_INT  ISRNumber=32  NumEventsToServe=1  EventsList={'on','EOC event','1';'off','Overflow event','2';'off','Custom event','3'}  SelectedEvents={'event1'}  TaskPriority=25  DisablePreemption=on  ClearInterruptFlagsAtEndOfEvent=on  InterruptDefinitionFile=$(TARGET_ROOT)/registry/interrupts/F2837xS_interrupts.xml  HardwareBoard=F2837x  EnableSimPort=off
      settings: LibrarySourceBlock=c2000lib/Scheduling/Hardware Interrupt
  HWI_ECAP2_INT : svdschedulerlib/Hardware Interrupt v2  ISRGroup=ADC - Analog to Digital Converter  ISRName=ADCA1_INT  ISRNumber=32  NumEventsToServe=1  EventsList={'on','EOC event','1';'off','Overflow event','2';'off','Custom event','3'}  SelectedEvents={'event1'}  TaskPriority=25  DisablePreemption=on  ClearInterruptFlagsAtEndOfEvent=on  InterruptDefinitionFile=$(TARGET_ROOT)/registry/interrupts/F2837xS_interrupts.xml  HardwareBoard=F2837x  EnableSimPort=off
      settings: LibrarySourceBlock=c2000lib/Scheduling/Hardware Interrupt
  HWI_ECAP3_INT : svdschedulerlib/Hardware Interrupt v2  ISRGroup=ADC - Analog to Digital Converter  ISRName=ADCA1_INT  ISRNumber=32  NumEventsToServe=1  EventsList={'on','EOC event','1';'off','Overflow event','2';'off','Custom event','3'}  SelectedEvents={'event1'}  TaskPriority=25  DisablePreemption=on  ClearInterruptFlagsAtEndOfEvent=on  InterruptDefinitionFile=$(TARGET_ROOT)/registry/interrupts/F2837xS_interrupts.xml  HardwareBoard=F2837x  EnableSimPort=off
      settings: LibrarySourceBlock=c2000lib/Scheduling/Hardware Interrupt
  HWI_SCIA_RX_INT : svdschedulerlib/Hardware Interrupt v2  ISRGroup=ADC - Analog to Digital Converter  ISRName=ADCA1_INT  ISRNumber=32  NumEventsToServe=1  EventsList={'on','EOC event','1';'off','Overflow event','2';'off','Custom event','3'}  SelectedEvents={'event1'}  TaskPriority=50  DisablePreemption=on  ClearInterruptFlagsAtEndOfEvent=on  InterruptDefinitionFile=$(TARGET_ROOT)/registry/interrupts/F2837xS_interrupts.xml  HardwareBoard=F2837x  EnableSimPort=off
      settings: LibrarySourceBlock=c2000lib/Scheduling/Hardware Interrupt
  Mux : Mux  Inputs=5
  HW_INT : Outport  VectorParamsAs1DForOutWhenUnconnected=off
  wires:
  HWI_ADCB1_INT/1 -> Mux/1
  HWI_ECAP3_INT/1 -> Mux/5
  HWI_SCIA_RX_INT/1 -> Mux/2
  HWI_ECAP2_INT/1 -> Mux/4
  HWI_ECAP1_INT/1 -> Mux/3
  Mux/1 -> HW_INT/1

== system mcb_pmsm_foc_hall_f28379d_state_indicator/HW Interrupt/Simulation ==
  Function-Call Generator{,1,3..4} (4 alike) : simulink/Ports & Subsystems/Function-Call Generator  sample_time=T_pwm  numberOfIterations=1  DisallowWideOutput=off
  Function-Call Generator2 : simulink/Ports & Subsystems/Function-Call Generator  sample_time=0.1  numberOfIterations=1  DisallowWideOutput=off
  Mux : Mux  Inputs=5
  HW_INT : Outport  VectorParamsAs1DForOutWhenUnconnected=off
  wires:
  Function-Call Generator2/1 -> Mux/2
  Mux/1 -> HW_INT/1
  Function-Call Generator/1 -> Mux/1
  Function-Call Generator1/1 -> Mux/3
  Function-Call Generator3/1 -> Mux/4
  Function-Call Generator4/1 -> Mux/5

== system mcb_pmsm_foc_hall_f28379d_state_indicator/Hall Sensor A/Capture Event Selection ==
  Hall State : Inport
  If : If  IfExpression=(u1 == 5 | u1 == 3)
  Merge : Merge
  Output 0 : Subsystem  TreatAsAtomicUnit=on
  Output 1 : Subsystem  TreatAsAtomicUnit=on
  Capture Event Select : Outport
  wires:
  Hall State/1 -> If/1
  Merge/1 -> Capture Event Select/1
  Output 0/1(Out1) -> Merge/2
  If/2 -> Output 0/Action
  If/1 -> Output 1/Action
  Output 1/1(Out1) -> Merge/1

== system mcb_pmsm_foc_hall_f28379d_state_indicator/Hall Sensor A/HallValidity ==
  CodeGen : Subsystem  VariantControl=(codegen)
  Sim : Subsystem  VariantControl=(sim)
  Out1 : Outport

== system mcb_pmsm_foc_hall_f28379d_state_indicator/Hall Sensor A/eCAP ==
  Code generation : Subsystem  VariantControl=(codegen)
  Simulation : Subsystem  VariantControl=(sim)
  eCAP_Out : Outport

== system mcb_pmsm_foc_hall_f28379d_state_indicator/Hall Sensor B/Capture Event Selection ==
  Hall State : Inport
  If : If  IfExpression=(u1 == 3 | u1 == 6)
  Merge : Merge
  Output 0 : Subsystem  TreatAsAtomicUnit=on
  Output 1 : Subsystem  TreatAsAtomicUnit=on
  Capture Event Select : Outport
  wires:
  Output 1/1(Out1) -> Merge/1
  Output 0/1(Out1) -> Merge/2
  If/2 -> Output 0/Action
  If/1 -> Output 1/Action
  Hall State/1 -> If/1
  Merge/1 -> Capture Event Select/1

== system mcb_pmsm_foc_hall_f28379d_state_indicator/Hall Sensor B/HallValidity ==
  CodeGen : Subsystem  VariantControl=(codegen)
  Sim : Subsystem  VariantControl=(sim)
  Out1 : Outport

== system mcb_pmsm_foc_hall_f28379d_state_indicator/Hall Sensor B/eCAP ==
  Code generation : Subsystem  VariantControl=(codegen)
  Simulation : Subsystem  VariantControl=(sim)
  eCAP_Out : Outport

== system mcb_pmsm_foc_hall_f28379d_state_indicator/Hall Sensor C/Capture Event Selection ==
  Hall State : Inport
  If : If  IfExpression=(u1 == 5 | u1 == 6)
  Merge : Merge
  Output 0 : Subsystem  TreatAsAtomicUnit=on
  Output 1 : Subsystem  TreatAsAtomicUnit=on
  Capture Event Select : Outport
  wires:
  Output 1/1(Out1) -> Merge/1
  Output 0/1(Out1) -> Merge/2
  If/2 -> Output 0/Action
  If/1 -> Output 1/Action
  Hall State/1 -> If/1
  Merge/1 -> Capture Event Select/1

== system mcb_pmsm_foc_hall_f28379d_state_indicator/Hall Sensor C/HallValidity ==
  CodeGen : Subsystem  VariantControl=(codegen)
  Sim : Subsystem  VariantControl=(sim)
  Out1 : Outport

== system mcb_pmsm_foc_hall_f28379d_state_indicator/Hall Sensor C/eCAP ==
  Code generation : Subsystem  VariantControl=(codegen)
  Simulation : Subsystem  VariantControl=(sim)
  eCAP_Out : Outport

== system mcb_pmsm_foc_hall_f28379d_state_indicator/Hardware Init/Variant Subsystem ==
  In1 : Inport
  Code Generation : Subsystem  VariantControl=(codegen)
  Simulation : Subsystem  VariantControl=(sim)

== system mcb_pmsm_foc_hall_f28379d_state_indicator/Heartbeat LED/Heartbeat LED ==
  In1 : Inport
  Code generation : Subsystem  VariantControl=(codegen)
  Simulation : Subsystem  VariantControl=(sim)

== system mcb_pmsm_foc_hall_f28379d_state_indicator/Inverter and Motor - Plant Model/Codegeneration ==
  Duty_Cycles : Inport
  Ground : Ground
  Ground1 : Ground
  Terminator : Terminator
  Iab_fb_Sim : Outport  VectorParamsAs1DForOutWhenUnconnected=off
  Pos_fb_Sim : Outport  Port=2  VectorParamsAs1DForOutWhenUnconnected=off
  wires:
  Duty_Cycles/1 -> Terminator/1
  Ground/1 -> Iab_fb_Sim/1
  Ground1/1 -> Pos_fb_Sim/1

== system mcb_pmsm_foc_hall_f28379d_state_indicator/Inverter and Motor - Plant Model/Simulation ==
  Duty_Cycles : Inport
  Inverter : Subsystem
  Load_Profile (Torque) : Subsystem
  RT1 : RateTransition  Deterministic=off  OutPortSampleTime=Ts_simulink
  RT3 : RateTransition  Deterministic=off  OutPortSampleTime=Ts_simulink
  Rate Transition : RateTransition  Deterministic=off  OutPortSampleTime=Ts_motor
  Rate Transition1 : RateTransition  Deterministic=off  OutPortSampleTime=Ts_motor
  Sensor_Measurements : Subsystem
  Surface Mount PMSM : autolibpmsmexterior/Surface Mount PMSM  port_config=Torque  sim_type=Discrete  Ts=Ts_motor  P=pmsm.p  Rs=pmsm.Rs + inverter.R_board  Ldq_=pmsm.Ld  KConstText=Permanent flux linkage constant (lambda_pm):  lambda_pm=pmsm.FluxPM  Ke=159.9771  Kt=1.323  mechanical=[pmsm.J, pmsm.B, 0]  idq0=[0 0]  theta_init=0  omega_init=0  KConst=pmsm.FluxPM  lambda_pm_calc=pmsm.FluxPM  RefBlkName='autolibpmsmexterior/Surface Mount PMSM'  aMode=5  Ldq="[0.0002      0.0002]"
  Terminator : Terminator
  Iab_fb_Sim : Outport  VectorParamsAs1DForOutWhenUnconnected=off
  Pos_fb_Sim : Outport  Port=2  VectorParamsAs1DForOutWhenUnconnected=off
  wires:
  Sensor_Measurements/1(Iab meas ADC) -> Iab_fb_Sim/1
  Sensor_Measurements/2(Pos_mech) -> Pos_fb_Sim/1
  RT3/1 -> Sensor_Measurements/1(Info)
  Rate Transition1/1 -> Surface Mount PMSM/1
  RT1/1 -> Sensor_Measurements/2(Iab meas)
  Load_Profile (Torque)/1(Load_Trq) -> Rate Transition1/1
  Surface Mount PMSM/3 -> Terminator/1
  Duty_Cycles/1 -> Inverter/1(Duty_abc)
  Surface Mount PMSM/2 -> RT1/1  "Iabc"
  Surface Mount PMSM/1 -> RT3/1
  Rate Transition/1 -> Surface Mount PMSM/2
  Inverter/1(Vabc) -> Rate Transition/1

== system mcb_pmsm_foc_hall_f28379d_state_indicator/Serial Receive/Data_Conditioning_Rx ==
  In1 : Inport
  Data_Type_Fixed_Point : Subsystem  VariantControl=~isequal(dataType, 'single')
  Data_Type_Float : Subsystem  VariantControl=isequal(dataType, 'single')
  Desired Speed : Outport
  Out2 : Outport  Port=2

== system mcb_pmsm_foc_hall_f28379d_state_indicator/Serial Receive/SCI_Rx ==
  Code Generation : Subsystem  Variant=on  VariantControl=(codegen)
  Simulation : Subsystem  VariantControl=(sim)
  Data : Outport

== system mcb_pmsm_foc_hall_f28379d_state_indicator/Serial Receive/unParse ==
  Data : Inport
  Bitwise Operator : simulink/Logic and Bit Operations/Bitwise Operator  logicop=AND  UseBitMask=on  BitMask=hex2dec('0001')  BitMaskRealWorld=Stored Integer
  Bitwise Operator1 : simulink/Logic and Bit Operations/Bitwise Operator  logicop=AND  UseBitMask=on  BitMask=hex2dec('00F0')  BitMaskRealWorld=Stored Integer
  Data Type Conversion3 : DataTypeConversion  OutDataTypeStr=boolean  RndMeth=Simplest  SaturateOnIntegerOverflow=off
  Data Type Conversion4 : DataTypeConversion  OutDataTypeStr=uint16  RndMeth=Simplest  SaturateOnIntegerOverflow=off
  Shift Arithmetic1 : ArithShift  BitShiftNumber=4
  Enable_PWM : Outport
  Debug_signals : Outport  Port=2
  wires:
  Bitwise Operator1/1 -> Shift Arithmetic1/1
  Data/1 -> Bitwise Operator/1, Bitwise Operator1/1
  Bitwise Operator/1 -> Data Type Conversion3/1
  Data Type Conversion4/1 -> Debug_signals/1
  Shift Arithmetic1/1 -> Data Type Conversion4/1
  Data Type Conversion3/1 -> Enable_PWM/1

== system mcb_pmsm_foc_hall_f28379d_state_indicator/Speed Control/PI_Controller_Speed ==
  N_ref : Inport
  N_fb : Inport  Port=2
  Data Store Read2 : DataStoreRead  DataStoreName=Enable  IndexOptions=Index vector (dialog)  Indices=1  OutputSizes=1
  Discrete PI Controller with anti-windup & reset : slpidlib/PID Controller  Controller=PI  Form=Parallel  TimeDomain=Discrete-time  UseExternalTs=off  SampleTime=-1  IntegratorMethod=Forward Euler  FilterMethod=Forward Euler  ControllerParametersSource=external  P=1  I=1  UseKiTs=on  D=0  N=100  UseFilter=on  TunerSelectOption=Transfer Function Based (PID Tuner App)  InitialConditionSource=external  InitialConditionForIntegrator=0  InitialConditionForFilter=0  DifferentiatorICPrevScaledInput=0  ExternalReset=level  TrackingMode=off  Kt=1  LimitOutput=on  SatLimitsSource=internal  UpperSaturationLimit=1  LowerSaturationLimit=-1  LinearizeAsGain=on  AntiWindupMode=clamping  Kb=1  LimitIntegrator=off  UpperIntegratorSaturationLimit=inf  LowerIntegratorSaturationLimit=-inf  RndMeth=Simplest  POutMin=[]  POutMax=[]  IOutMin=[]  IOutMax=[]  DOutMin=[]  DOutMax=[]  NOutMin=[]  NOutMax=[]  SumOutMin=[]  SumOutMax=[]  SaturationOutDataTypeStr=Inherit: Inherit via back propagation  SaturationOutMin=[]  SaturationOutMax=[]  PParamMin=[]  PParamMax=[]  IParamMin=[]  IParamMax=[]  DParamMin=[]  DParamMax=[]  NParamMin=[]  NParamMax=[]  KbParamMin=[]  KbParamMax=[]  KtParamMin=[]  KtParamMax=[]  KbOutMin=[]  KbOutMax=[]  KtOutMin=[]  KtOutMax=[]  IntegratorOutMin=[]  IntegratorOutMax=[]  FilterOutMin=[]  FilterOutMax=[]  SumI1OutMin=[]  SumI1OutMax=[]  SumI2OutMin=[]  SumI2OutMax=[]  SumI3OutMin=[]  SumI3OutMax=[]  SumI4OutMin=[]  SumI4OutMax=[]  SumDOutMin=[]  SumDOutMax=[]  DifferentiatorOutMin=[]  DifferentiatorOutMax=[]  FilterDiffOutCoefMin=[]  FilterDiffOutCoefMax=[]  ReciprocalOutMin=[]  ReciprocalOutMax=[]  SumDenOutMin=[]  SumDenOutMax=[]  SumNumOutMin=[]  SumNumOutMax=[]  DivideOutMin=[]  DivideOutMax=[]  UdiffTsProdOutMin=[]  UdiffTsProdOutMax=[]  NTsProdOutMin=[]  NTsProdOutMax=[]  UintegralTsProdOutMin=[]  UintegralTsProdOutMax=[]  UngainTsProdOutMin=[]  UngainTsProdOutMax=[]  ClampingZeroOutDataTypeStr=Inherit: Inherit via back propagation  ClampingZeroOutMin=[]  ClampingZeroOutMax=[]  FilterDenConstantOutDataTypeStr=Inherit: Inherit via back propagation  FilterDenConstantOutMin=[]  FilterDenConstantOutMax=[]  PCopyOutDataTypeStr=Inherit: Inherit via back propagation  PCopyOutMin=[]  PCopyOutMax=[]  NCopyOutDataTypeStr=Inherit: Inherit via back propagation  NCopyOutMin=[]  NCopyOutMax=[]  IntegratorContinuousStateAttributes=''  IntegratorStateMustResolveToSignalObject=off  IntegratorRTWStateStorageClass=Auto  FilterContinuousStateAttributes=''  FilterStateMustResolveToSignalObject=off  FilterRTWStateStorageClass=Auto  ParallelPVariant=ExternalParameters  IdealPVariant=Disabled  IVariant=ExternalParameters  DVariant=Disabled  IntegratorVariant=Discrete  SatVariant=Enabled  AWVariant=DiscClampingParallel  PCopyVariant=Disabled  TRVariant=Disabled  FdbkBlocksVariant=Forward  IdealPFdbkVariant=Disabled  SatFdbkVariant=Disabled  DerivativeFilterVariant=Disabled  NVariant=Disabled  NCopyVariant=Disabled_SignalSpec  FilterICVariant=Disabled  IntegratorICVariant=ExternalICs  ExternalResetVariant=ExternalReset  TRSumVariant=Passthrough  SumFdbkVariant=Disabled  SumVariant=Sum_PI  TsampFilterVariant=InternalTs  TsampNgainVariant=Passthrough  TsampIntegralVariant=Disabled_SignalSpec  ExternalSaturationOutDataTypeStr=Inherit: Same as second input
      settings: LibrarySourceBlock=mcbcontrolslib/PI Controller
  Ki1 : Constant  Value=PI_params.Ki_speed*Ts_speed  OutDataTypeStr=dataType  SampleTime=-1
  Ki2 : Constant  Value=0  OutDataTypeStr=dataType  SampleTime=-1
  Kp1 : Constant  Value=PI_params.Kp_speed  OutDataTypeStr=dataType  SampleTime=-1
  Logical Operator : Logic  Operator=NOT  IconShape=distinctive  AllPortsSameDT=off  OutDataTypeStr=boolean
  Sum : Sum  Inputs=|+-  RndMeth=Round
  Zero_Cancellation : mcbcontrolslib/IIR Filter  VariantControl=Low Pass Filter  VariantSelect=Low-pass  Filter_constant=0.01*(Ts_speed/Ts)  advancedSettings=off  Ts=50e-6  cutOff_freq=353.6777
  Iq_ref : Outport  VectorParamsAs1DForOutWhenUnconnected=off
  wires:
  Discrete PI Controller with anti-windup & reset/1 -> Iq_ref/1
  Ki1/1 -> Discrete PI Controller with anti-windup & reset/3
  Kp1/1 -> Discrete PI Controller with anti-windup & reset/2
  N_fb/1 -> Sum/2
  N_ref/1 -> Zero_Cancellation/1
  Logical Operator/1 -> Discrete PI Controller with anti-windup & reset/4
  Ki2/1 -> Discrete PI Controller with anti-windup & reset/5
  Sum/1 -> Discrete PI Controller with anti-windup & reset/1
  Data Store Read2/1 -> Logical Operator/1
  Zero_Cancellation/1 -> Sum/1
